simulink model "obs_pert_sin"  (R2025b)
settings: Solver=VariableStepAuto  StartTime=0.0  StopTime=500  RelTol=1e-3
values from neighbouring files (symbols this model uses):
  A = [0 1 0 0 ... (first row only)    [porte_avion.m]
  A_obs2 = [A           E2 ... (first row only)    [porte_avion.m]
  B = [0 ... (first row only)    [porte_avion.m]
  B_obs2 = [B; 0; 0]    [porte_avion.m]
  C2 = [1 0 0 0 ... (first row only)    [porte_avion.m]
  C_obs2 = [C2 zeros(2, 2)]    [porte_avion.m]
  D2 = [0 ... (first row only)    [porte_avion.m]
  H = -pinv((C) * ((A - B*K) \ B))    [porte_avion.m]
  K = place(A, B, poles_cmd)    [porte_avion.m]
  Ki = -2000    [porte_avion.m]
  L_obs2 = place(A_obs2', C_obs2', [-2, -2.5, -3, -3.5, -4, -4.5])'    [porte_avion.m]
  r = 0    [porte_avion.m]
  X_0 = [x_0 ... (first row only)    [porte_avion.m]
settings Model: Creator=vikfo  LastModifiedBy=victor

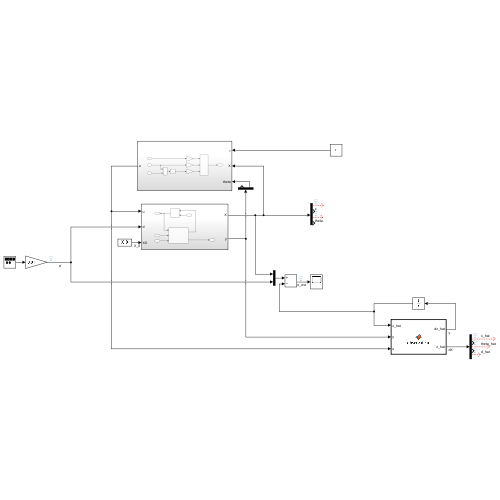
[thumbnail: Simulink's stored preview of the top-level diagram]
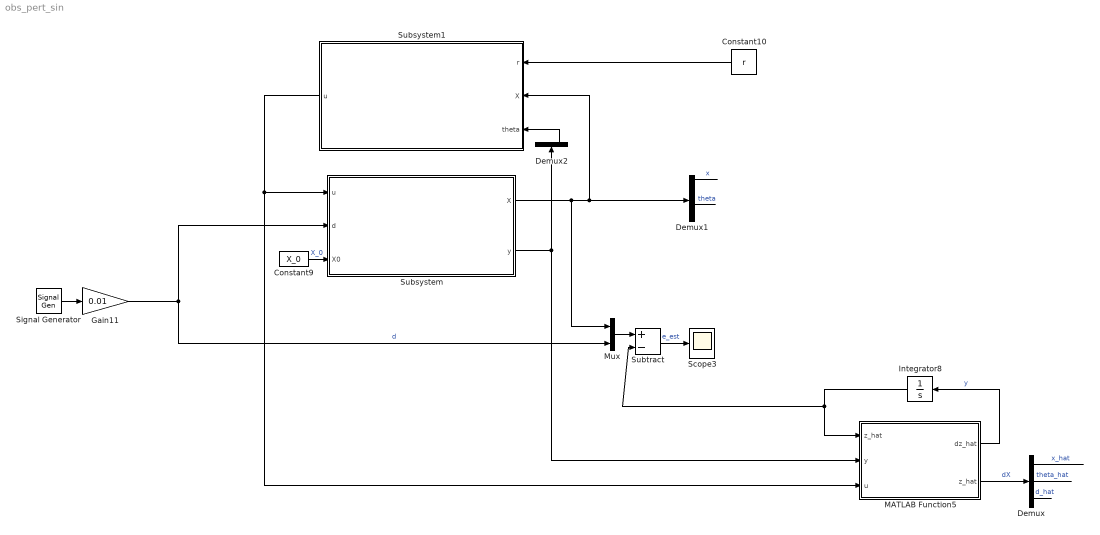
== system obs_pert_sin ==
  Constant10 : Constant  Value=r
  Constant9 : Constant  Value=X_0
  Demux : Demux  Outputs=5
  Demux1 : Demux
  Demux2 : Demux  Outputs=2
  Gain11 : Gain  Gain=0.01
  Integrator8 : Integrator  InitialCondition=zeros(5, 1)
  MATLAB Function5 : MATLAB Function  TreatAsAtomicUnit=on
  Mux : Mux  Inputs=[4 1]
  Scope3 : Scope
      settings: ActiveDisplayYMinimum=-1.369875447599938  ActiveDisplayYMaximum=0.62027967456851218  DataLoggingVariableName=ScopeData3
  Signal Generator : SignalGenerator  Frequency=0.2  Units=rad/sec
  Subsystem : Subsystem
  Subsystem1 : Subsystem
  Subtract : Sum  Inputs=+-
  wires:
  Gain11/1 -> Mux/2, Subsystem/2(d)  "d"
  MATLAB Function5/1(dz_hat) -> Integrator8/1  "y"
  Integrator8/1 -> Subtract/2, MATLAB Function5/1("z_hat ")
  MATLAB Function5/2(z_hat) -> Demux/1  "dX"
  Demux/5 -> ?  "d_hat"
  Demux/1 -> ?  "x_hat"
  Demux/3 -> ?  "theta_hat"
  Demux1/1 -> ?  "x"
  Demux1/3 -> ?  "theta"
  Mux/1 -> Subtract/1
  Subtract/1 -> Scope3/1  "e_est"
  Signal Generator/1 -> Gain11/1
  Subsystem/2(y) -> Demux2/1, MATLAB Function5/2(y)
  Subsystem/1(X) -> Demux1/1, Subsystem1/2(X), Mux/1
  Constant9/1 -> Subsystem/3(X0)  "X_0"
  Subsystem1/1(u) -> MATLAB Function5/3(u), Subsystem/1(u)
  Constant10/1 -> Subsystem1/1(r)
  Demux2/2 -> Subsystem1/3(theta)

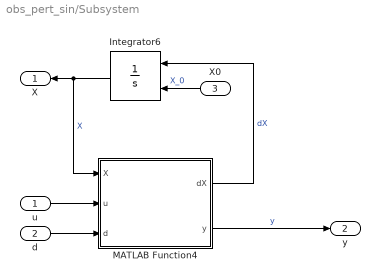
== system obs_pert_sin/Subsystem ==
  u : Inport
  d : Inport  Port=2
  X0 : Inport  Port=3
  Integrator6 : Integrator  InitialConditionSource=external
  MATLAB Function4 : MATLAB Function  TreatAsAtomicUnit=on
  X : Outport
  y : Outport  Port=2
  wires:
  MATLAB Function4/2(y) -> y/1  "y"
  X0/1 -> Integrator6/2  "X_0"
  Integrator6/1 -> MATLAB Function4/1(X), X/1  "X"
  MATLAB Function4/1(dX) -> Integrator6/1  "dX"
  d/1 -> MATLAB Function4/3(d)
  u/1 -> MATLAB Function4/2(u)

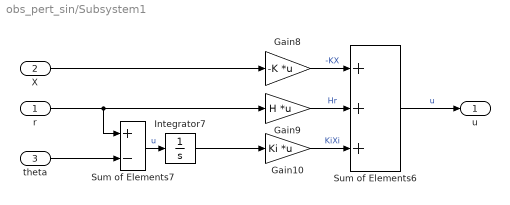
== system obs_pert_sin/Subsystem1 ==
  r : Inport
  X : Inport  Port=2
  theta : Inport  Port=3
  Gain10 : Gain  Gain=Ki  Multiplication=Matrix(K*u)
  Gain8 : Gain  Gain=-K  Multiplication=Matrix(K*u)
  Gain9 : Gain  Gain=H  Multiplication=Matrix(K*u)
  Integrator7 : Integrator
  Sum of Elements6 : Sum  Inputs=+++
  Sum of Elements7 : Sum  Inputs=+-
  u : Outport
  wires:
  Gain8/1 -> Sum of Elements6/1  "-KX"
  Gain9/1 -> Sum of Elements6/2  "Hr"
  Gain10/1 -> Sum of Elements6/3  "KiXi"
  theta/1 -> Sum of Elements7/2
  X/1 -> Gain8/1
  Sum of Elements7/1 -> Integrator7/1  "u"
  Integrator7/1 -> Gain10/1
  r/1 -> Sum of Elements7/1, Gain9/1
  Sum of Elements6/1 -> u/1  "u"

== matlab function obs_pert_sin/Subsystem/MATLAB Function4 ==
  data: X input; u input; d input; dX output; y output; A parameter; B parameter; C2 parameter; D2 parameter; E parameter
function [dX, y]= porte_avion_dyn(X, u, d, A, B, C2, D2, E)
dX = A*X + B*u + E*d;
y = C2*X + D2*u;
end

== matlab function obs_pert_sin/MATLAB Function5 ==
  data: dz_hat output; z_hat input; y input; u input; A_obs2 parameter; z_hat output; B_obs2 parameter; C_obs2 parameter; L_obs2 parameter
function [dz_hat, z_hat]= observateur(z_hat, y, u, A_obs2, B_obs2, C_obs2, L_obs2)
dz_hat = zeros(6, 1);
dz_hat = A_obs2*z_hat + B_obs2*u + L_obs2*(y - C_obs2*z_hat);
end
